simulink model "AXI_testIP"  (R2020b)
settings: Solver=FixedStepDiscrete  StartTime=0.0  StopTime=10.0  RelTol=1e-3
settings Model: DataTypeOverride=Off  Creator=ts  LastModifiedBy=ts
settings DataIOCC: LimitDataPoints=on  SaveOutput=off  SaveTime=off
settings OptimizationCC: BlockReduction=off  ConditionallyExecuteInputs=off  DefaultParameterBehavior=Inlined  LifeSpan=inf
settings DebuggingCC: AlgebraicLoopMsg=error  SingleTaskRateTransMsg=error  AllowSymbolicDim=off  StrictBusMsg=ErrorOnBusTreatedAsVector  SFUnexpectedBacktrackingDiag=warning  SFNoUnconditionalDefaultTransitionDiag=warning  SFExecutionAtInitializationDiag=none  ArithmeticOperatorsInVariantConditions=warning
settings HardwareCC: ProdBitPerPointer=32  ProdBitPerSizeT=32  ProdBitPerPtrDiffT=32  ProdLargestAtomicFloat=None  ProdIntDivRoundTo=Undefined  ProdEndianess=Unspecified  ProdWordSize=32  ProdHWDeviceType=ASIC/FPGA->ASIC/FPGA  ProdEqTarget=off
settings SFSimCC: SimUseLocalCustomCode=off  CustomCodeUndefinedFunction=UseInterfaceOnly
settings RTWCC: RTWUseLocalCustomCode=off
settings CodeAppCC: StateflowObjectComments=on
settings GRTTargetCC: TargetLangStandard=C89/C90 (ANSI)
settings ConfigComp: CovScope=ReferencedModels  CovMetricSettings=dw  CovSaveCumulativeToWorkspaceVar=on  CovSaveSingleToWorkspaceVar=on  CovExternalEMLEnable=off  CovSFcnEnable=off

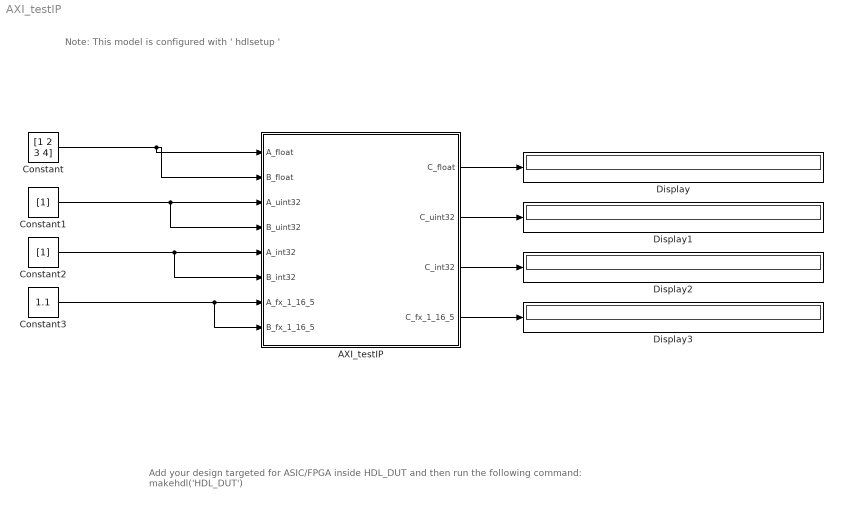
== system AXI_testIP ==
  note: Note: This model is configured with ' hdlsetup '
  note: Add your design targeted for ASIC/FPGA inside HDL_DUT and then run the following command:
      | makehdl('HDL_DUT')
  AXI_testIP : Subsystem  TreatAsAtomicUnit=on
  Constant : Constant  Value=[1 2 3 4]  OutDataTypeStr=single  SampleTime=-1
  Constant1 : Constant  Value=[1]  OutDataTypeStr=uint32  SampleTime=-1
  Constant2 : Constant  Value=[1]  OutDataTypeStr=int32  SampleTime=-1
  Constant3 : Constant  Value=1.1  OutDataTypeStr=fixdt(1,16,5)  SampleTime=-1
  Display{,1..3} (4 alike) : Display
  wires:
  Constant/1 -> AXI_testIP/2(B_float), AXI_testIP/1(A_float)
  AXI_testIP/1(C_float) -> Display/1
  Constant1/1 -> AXI_testIP/4(B_uint32), AXI_testIP/3(A_uint32)
  AXI_testIP/2(C_uint32) -> Display1/1
  AXI_testIP/3(C_int32) -> Display2/1
  AXI_testIP/4(C_fx_1_16_5) -> Display3/1
  Constant2/1 -> AXI_testIP/6(B_int32), AXI_testIP/5(A_int32)
  Constant3/1 -> AXI_testIP/8(B_fx_1_16_5), AXI_testIP/7(A_fx_1_16_5)

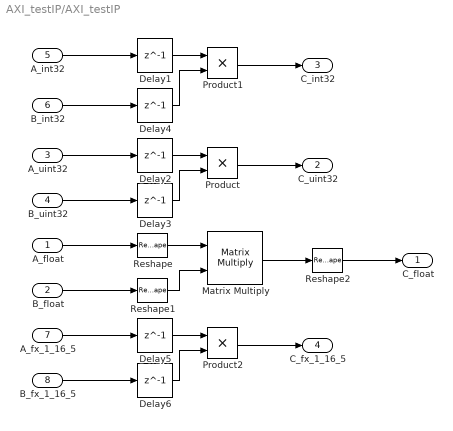
== system AXI_testIP/AXI_testIP ==
  A_float : Inport
  B_float : Inport  Port=2
  A_uint32 : Inport  Port=3
  B_uint32 : Inport  Port=4
  A_int32 : Inport  Port=5
  B_int32 : Inport  Port=6
  A_fx_1_16_5 : Inport  Port=7
  B_fx_1_16_5 : Inport  Port=8
  Delay{1..6} (6 alike) : Delay  DelayLength=1
  Matrix Multiply : Product  Multiplication=Matrix(*)
  Product : Product  OutDataTypeStr=Inherit: Same as first input
  Product1 : Product  OutDataTypeStr=Inherit: Same as first input
  Product2 : Product  OutDataTypeStr=Inherit: Same as first input
  Reshape : Reshape  OutputDimensionality=Customize  OutputDimensions=[2,2]
  Reshape1 : Reshape  OutputDimensionality=Customize  OutputDimensions=[2,2]
  Reshape2 : Reshape
  C_float : Outport  VectorParamsAs1DForOutWhenUnconnected=off
  C_uint32 : Outport  Port=2  VectorParamsAs1DForOutWhenUnconnected=off
  C_int32 : Outport  Port=3  VectorParamsAs1DForOutWhenUnconnected=off
  C_fx_1_16_5 : Outport  Port=4  VectorParamsAs1DForOutWhenUnconnected=off
  wires:
  Matrix Multiply/1 -> Reshape2/1
  Product/1 -> C_uint32/1
  Product2/1 -> C_fx_1_16_5/1
  Delay2/1 -> Product/1
  B_int32/1 -> Delay4/1
  A_int32/1 -> Delay1/1
  Delay5/1 -> Product2/1
  A_fx_1_16_5/1 -> Delay5/1
  Product1/1 -> C_int32/1
  Delay6/1 -> Product2/2
  B_fx_1_16_5/1 -> Delay6/1
  Delay4/1 -> Product1/2
  Reshape2/1 -> C_float/1
  Delay1/1 -> Product1/1
  Delay3/1 -> Product/2
  A_float/1 -> Reshape/1
  B_float/1 -> Reshape1/1
  Reshape/1 -> Matrix Multiply/1
  A_uint32/1 -> Delay2/1
  Reshape1/1 -> Matrix Multiply/2
  B_uint32/1 -> Delay3/1
